simulink model "CC_Flight_Simulation"  (R2024b)
settings: Solver=ode45  StartTime=0.0  StopTime=60  MaxStep=0.002  RelTol=1e-5
values from neighbouring files (symbols this model uses):
  location = [10 43.47 -80.54]    [barrowman.mat]
libraries: simulink_extras x4, aerolibanim x1, dspindex x1, sharedtransform x1
settings Model: Creator=bruno  LastModifiedBy=finnb
settings SolverCC: AlgebraicLoopSolver=TrustRegion
settings OptimizationCC: LifeSpan=inf
settings DebuggingCC: UnconnectedInputMsg=warning  UnconnectedOutputMsg=warning  UnconnectedLineMsg=warning  ArithmeticOperatorsInVariantConditions=warning
settings ModelReferenceCC: EnableRefExpFcnMdlSchedulingChecks=on
settings SFSimCC: CustomCodeUndefinedFunction=UseInterfaceOnly  SimTargetLang=C++
settings RTWCC: GPUComputeCapability=3.5
settings CodeAppCC: StateflowObjectComments=on
settings SimscapeCC: SimscapeNormalizeSystem=off

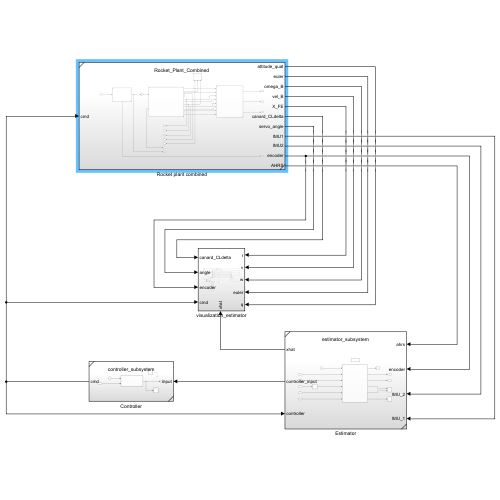
[thumbnail: Simulink's stored preview of the top-level diagram]
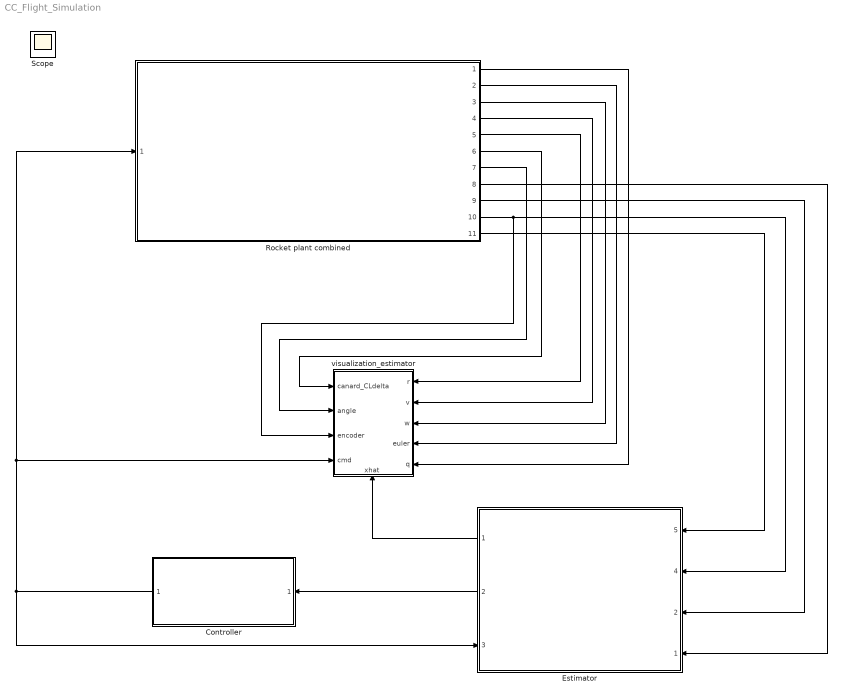
== system CC_Flight_Simulation ==
  Controller : Subsystem  ReferencedSubsystem=controller_subsystem
  Estimator : Subsystem  ReferencedSubsystem=estimator_subsystem
      settings: PortSchema="{\"entries\":[{\"content\":{\"sides\":[{\"content\":{\"connectorIds\":[\"In5\",\"In4\",\"In2\",\"In1\"]},\"type\":\"ConnectorPlacement.EquallySpacedRectSide\",\"uuid\":\"3a8674be-3010-4d68-a33c-3eead0b8fa7c\"},{\"content\":{\"connectorIds\":[\"Out1\",\"Out2\",\"In3\"],\"side\":\"RIGHT\"},\"type\":\"ConnectorPlacement.EquallySpacedRectSide\",\"uuid\":\"adad2a77-0efa-48c4-a551-5f502a84ce9d\"},{\"content\":{\"side\":\"TOP\"},\"type\":\"ConnectorPlacement.EquallySpacedRectSide\",\"uuid\":\"86d43adf-3710-4d07-a3fc-1076e1b690c3\"}]},\"type\":\"ConnectorPlacement.EquallySpacedConnector\",\"uuid\":\"03723af2-c1ac-4c1d-a4bb-0b905c3a6fdb\"}],\"packageUris\":[\"http://schema.mathworks.com/mf0/Connector/R2020b\"],\"version\":\"1.0\"}"
  Rocket plant combined : Subsystem  ReferencedSubsystem=Rocket_Plant_Combined
  visualization_estimator : Subsystem
      settings: PortSchema="{\"entries\":[{\"content\":{\"sides\":[{\"content\":{\"connectorIds\":[\"In1\",\"In2\",\"In3\",\"In4\",\"In5\"]},\"type\":\"ConnectorPlacement.EquallySpacedRectSide\",\"uuid\":\"dc5fb855-67c6-44f2-b840-f485865d62e2\"},{\"content\":{\"connectorIds\":[\"In7\",\"In8\",\"In9\",\"In10\"],\"side\":\"RIGHT\"},\"type\":\"ConnectorPlacement.EquallySpacedRectSide\",\"uuid\":\"f011a5d6-ba81-4cae-9458-00e11c499556\"},{\"content\":{\"side\":\"TOP\"},\"type\":\"ConnectorPlacement.EquallySpacedRectSide\",\"uuid\":\"2cb02a95-4340-4437-bf5a-0250095828b1\"},{\"content\":{\"connectorIds\":[\"In6\"],\"side\":\"BOTTOM\"},\"type\":\"ConnectorPlacement.EquallySpacedRectSide\",\"uuid\":\"f99cf30a-31eb-400e-ba65-b3afbbabbc8d\"}]},\"type\":\"ConnectorPlacement.EquallySpacedConnector\",\"uuid\":\"1a89fa10-7481-4e31-a831-abb3dd053fbf\"}],\"packageUris\":[\"http://schema.mathworks.com/mf0/Connector/R2020b\"],\"version\":\"1.0\"}"
  Scope : Scope
  wires:
  Estimator/1 -> visualization_estimator/6(xhat)
  Controller/1 -> Estimator/3, Rocket plant combined/1, visualization_estimator/10(cmd)
  Estimator/2 -> Controller/1
  Rocket plant combined/10 -> visualization_estimator/9(encoder), Estimator/4
  Rocket plant combined/1 -> visualization_estimator/5(q)
  Rocket plant combined/7 -> visualization_estimator/8(angle)
  Rocket plant combined/2 -> visualization_estimator/4(euler)
  Rocket plant combined/3 -> visualization_estimator/3(w)
  Rocket plant combined/4 -> visualization_estimator/2(v)
  Rocket plant combined/5 -> visualization_estimator/1(r)
  Rocket plant combined/11 -> Estimator/5
  Rocket plant combined/9 -> Estimator/2
  Rocket plant combined/8 -> Estimator/1
  Rocket plant combined/6 -> visualization_estimator/7(canard_CLdelta)

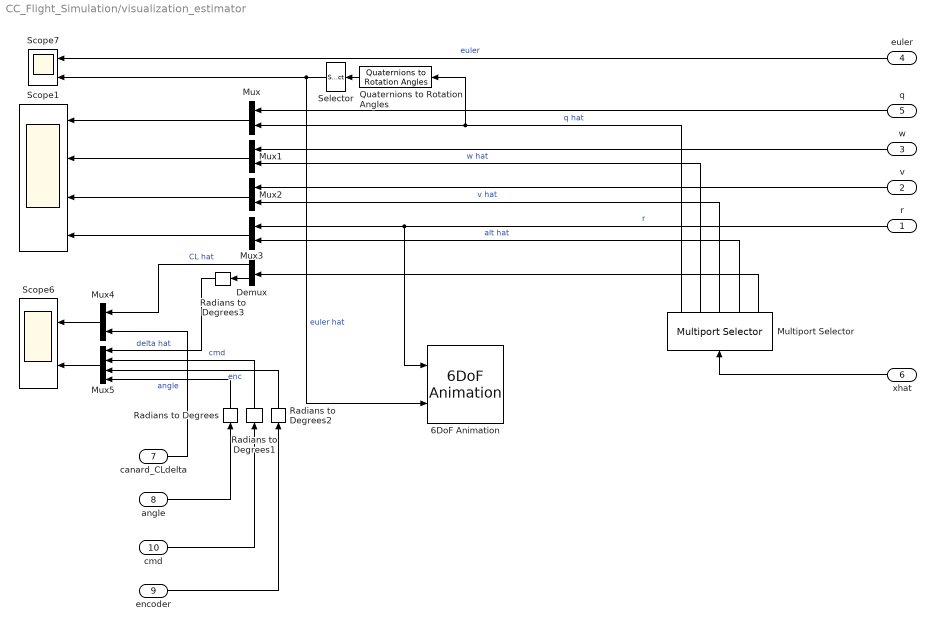
== system CC_Flight_Simulation/visualization_estimator ==
  r : Inport
  v : Inport  Port=2
  w : Inport  Port=3
  euler : Inport  Port=4
  q : Inport  Port=5
  xhat : Inport  Port=6
  canard_CLdelta : Inport  Port=7
  angle : Inport  Port=8
  encoder : Inport  Port=9
  cmd : Inport  Port=10
  6DoF Animation : aerolibanim/6DoF Animation  u1=[0 8000 -100 100 0 400]  u2=0.1  u3=5  u4=[location(1)-5 0 0]  u5=Fly alongside  u6=[0 100 0]  u7=10  u8=off
  Demux : Demux  Outputs=2
  Multiport Selector : dspindex/Multiport Selector  rowsOrCols=Rows  idxCellArray={ 1:4, 5:7, 8:10, 11, 12:13 }  idxErrMode=Clip Index
  Mux : Mux  Inputs=[4 4]
  Mux{1..4} (4 alike) : Mux  Inputs=2
  Mux5 : Mux
  Quaternions to Rotation Angles : sharedtransform/Quaternions to Rotation Angles  rotationOrder=ZYX  aMode=aMode
  Radians to Degrees{,1..3} (4 alike) : simulink_extras/Transformations/Radians to Degrees
  Scope1 : Scope  NumInputPorts=4
  Scope6 : Scope  NumInputPorts=2
  Scope7 : Scope  NumInputPorts=2
  Selector : Selector  InputPortWidth=3  IndexOptions=Index vector (dialog)  Indices=[3 2 1]  OutputSizes=1
  wires:
  Multiport Selector/5 -> Demux/1
  q/1 -> Mux/1
  w/1 -> Mux1/1
  Mux2/1 -> Scope1/3
  Multiport Selector/1 -> Quaternions to Rotation Angles/1, Mux/2  "q hat"
  xhat/1 -> Multiport Selector/1
  Multiport Selector/4 -> Mux3/2  "alt hat"
  Selector/1 -> 6DoF Animation/2, Scope7/2  "euler hat"
  Mux1/1 -> Scope1/2
  Multiport Selector/2 -> Mux1/2  "w hat"
  Multiport Selector/3 -> Mux2/2  "v hat"
  Mux/1 -> Scope1/1
  Mux3/1 -> Scope1/4
  v/1 -> Mux2/1
  r/1 -> Mux3/1, 6DoF Animation/1  "r"
  euler/1 -> Scope7/1  "euler"
  angle/1 -> Radians to Degrees/1
  cmd/1 -> Radians to Degrees1/1
  encoder/1 -> Radians to Degrees2/1
  Quaternions to Rotation Angles/1 -> Selector/1
  Radians to Degrees/1 -> Mux5/4  "angle"
  Radians to Degrees1/1 -> Mux5/2  "cmd"
  Radians to Degrees2/1 -> Mux5/3  "enc"
  Demux/2 -> Radians to Degrees3/1
  Demux/1 -> Mux4/1  "CL hat"
  Radians to Degrees3/1 -> Mux5/1  "delta hat"
  canard_CLdelta/1 -> Mux4/2
  Mux5/1 -> Scope6/2
  Mux4/1 -> Scope6/1
